simulink model "disturbance_height"  (R2016b)
settings: Solver=VariableStepAuto  StartTime=0.0  StopTime=10.0  RelTol=1e-3
undefined symbols (not defined in the file or in its folder): sample_time
settings Model: Creator=Jared  LastModifiedBy=Jared

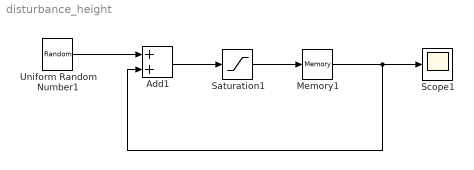
== system disturbance_height ==
  Add1 : Sum
  Memory1 : Memory  InheritSampleTime=on
  Saturation1 : Saturate  UpperLimit=0.4  LowerLimit=-0.4
  Scope1 : Scope
  Uniform Random Number1 : UniformRandomNumber  Minimum=-0.004  Maximum=0.004  Seed=20  SampleTime=sample_time
  wires:
  Saturation1/1 -> Memory1/1
  Add1/1 -> Saturation1/1
  Memory1/1 -> Add1/2, Scope1/1
  Uniform Random Number1/1 -> Add1/1
